simulink model "tutorial_picooz_acquire_extmode"  (R2025b)
settings: Solver=FixedStepDiscrete  StartTime=0.0  StopTime=60  FixedStep=0.001  RelTol=1e-3  EnableMultiTasking=on
undefined symbols (not defined in the file or in its folder): A0, ADC, D10, H0, Max, MaxPer, ms, ns, P1, P113, P59, Pin, PWM3_Trg1, Resol, us
libraries: MCHP_Blockset x8, simulink x5, dspsrcs4 x1, dspstat3 x1
(part 2 of 2)

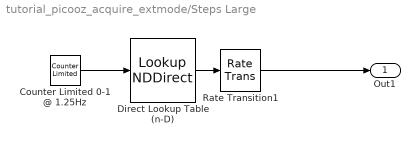
== system tutorial_picooz_acquire_extmode/Steps Large ==
  Counter Limited 0-1 @ 1.25Hz : simulink/Sources/Counter Limited  uplimit=19  tsamp=1
  Direct Lookup Table (n-D) : LookupNDDirect  NumberOfTableDimensions=1  Table=([0 0 10 20 30 40 50 60 70 80 70 60 50 40 30 20 10 0 50 80] / 50 ) - 1  TableDataTypeStr=single
  Rate Transition1 : RateTransition  Integrity=off  Deterministic=off
  Out1 : Outport
  wires:
  Direct Lookup Table (n-D)/1 -> Rate Transition1/1
  Counter Limited 0-1 @ 1.25Hz/1 -> Direct Lookup Table (n-D)/1
  Rate Transition1/1 -> Out1/1
